simulink model "AERO2_LQR_OBSERVADOR"  (R2025b)
settings: Solver=ode1  StartTime=0.0  StopTime=inf  FixedStep=0.002  RelTol=1e-3  EnableMultiTasking=on
values from neighbouring files (symbols this model uses):
  A_modelo = [0 0 1 0 ... (first row only)    [AERO2_LQR_OBSERVADOR.m]
  B_modelo = [0 0 ... (first row only)    [AERO2_LQR_OBSERVADOR.m]
  beta = double(solucion.beta)    [AERO2_LQR_OBSERVADOR.m]
  C = [1 0 0 0 ... (first row only)    [AERO2_LQR_OBSERVADOR.m]
  D = [0 0 ... (first row only)    [AERO2_LQR_OBSERVADOR.m]
  K_lqr = lqr(A_modelo, B_modelo, Q, R)    [AERO2_LQR_OBSERVADOR.m]
  l = double(solucion.l)    [AERO2_LQR_OBSERVADOR.m]
  m = double(solucion.m)    [AERO2_LQR_OBSERVADOR.m]
undefined symbols (not defined in the file or in its folder): HIL, qc_get_step_size
libraries: quarc_library x7
settings Model: ExtModeTrigDuration=10000  Creator=CPB0  LastModifiedBy=CPB0
settings SolverCC: AlgebraicLoopSolver=TrustRegion  PositivePriorityOrder=on
settings DataIOCC: ReturnWorkspaceOutputs=off
settings DebuggingCC: UnconnectedInputMsg=warning  UnconnectedOutputMsg=warning  UnconnectedLineMsg=warning  ArithmeticOperatorsInVariantConditions=warning
settings ModelReferenceCC: EnableRefExpFcnMdlSchedulingChecks=on
settings SFSimCC: SimUseLocalCustomCode=off  CustomCodeUndefinedFunction=UseInterfaceOnly
settings RTWCC: SystemTargetFile=quarc_win64.tlc  TemplateMakefile=quarc_default_tmf  RTWUseLocalCustomCode=off  Toolchain=QUARC win64 | nmake (64-bit Windows)  BuildConfiguration=Faster Runs  GPUComputeCapability=3.5  Description=QUARC Win64 Target Using Toolchain
settings CodeAppCC: StateflowObjectComments=on
settings STFCustomTargetCC: SystemTargetFile=quarc_win64.tlc  TargetLangStandard=C99 (ISO)  UseToolchainInfoCompliant=on
settings GRTTargetCC: ExtMode=on  ExtModeMexFile=quarc_comm  ParMdlRefBuildCompliant=off  CompOptLevelCompliant=off  CombineOutputUpdateFcns=off  MatFileLogging=off  CPPClassGenCompliant=off  GRTInterface=on
settings ConfigComp: CovMetricSettings=dswe

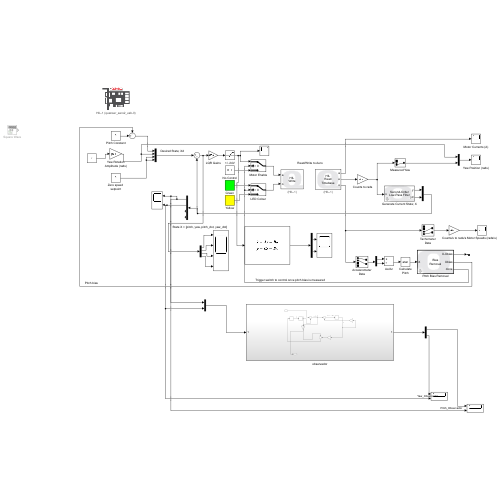
[thumbnail: Simulink's stored preview of the top-level diagram]
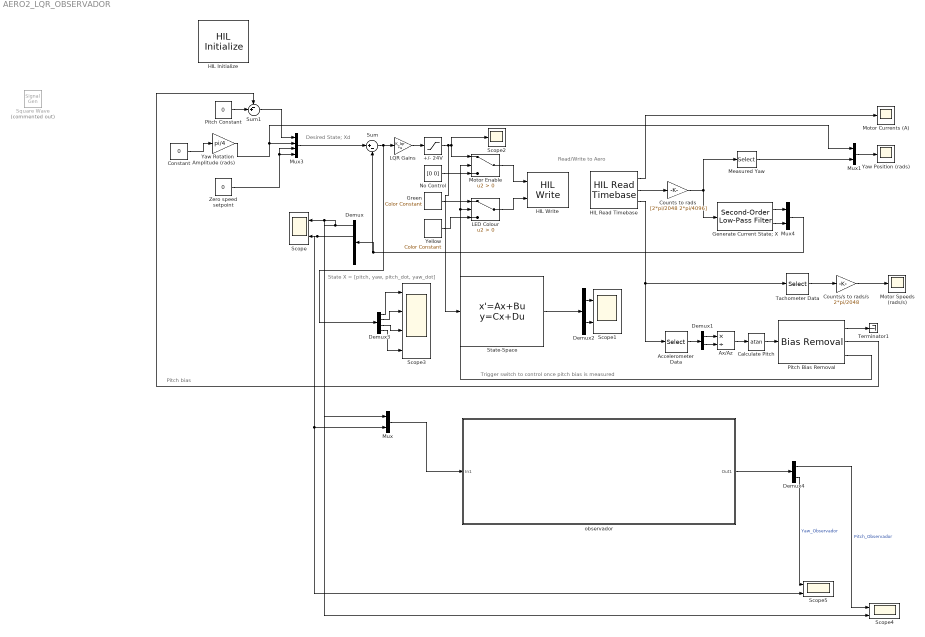
== system AERO2_LQR_OBSERVADOR ==
  note: Desired State; Xd
  note: Trigger switch to control once pitch bias is measured
  note: State X = [pitch, yaw, pitch_dot, yaw_dot]
  note: Pitch bias
  note: Read/Write to Aero
  +/- 24V : Saturate  UpperLimit=24  LowerLimit=-24
  Accelerometer Data : Selector  InputPortWidth=4  IndexOptions=Index vector (dialog)  Indices=[1 2]  OutputSizes=1
  Ax/Az : Product  Inputs=*/
  Calculate Pitch : Trigonometry  Operator=atan
  Constant : Constant  Value=0
  Counts to rads : Gain  Gain=[2*pi/2048 2*pi/4096]
  Counts/s to rads/s : Gain  Gain=2*pi/2048
  Demux : Demux
  Demux1 : Demux  Outputs=2
  Demux2 : Demux  Outputs=2
  Demux3 : Demux
  Demux4 : Demux  Outputs=2
  Generate Current State; X : quarc_library/Continuous/Second-Order Low-Pass Filter  params_source=Internal (dialog parameters)  input_width=50  input_zeta=0.8  input_init=0
  Green : quarc_library/Sources/Signals/Color Constant  color=[0 1 0]
      settings: SourceProductName=QUARC Targets
  HIL Initialize : quarc_library/Data Acquisition/Generic/Configuration/HIL Initialize  Priority=-99  object_name=HIL-1  board_type=quanser_aero2_usb  board_number=0  board_options=""  exclusive=off  active=off  hardware_clocks=[0]  clock_modes=[]  initial_clock_frequencies=[]  set_clock_params_at_start=off  set_clock_params_at_switch_in=off  set_clock_frequencies_at_start=off  set_clock_frequencies_at_switch_in=off  analog_input_channels=[0:1]  analog_input_configurations=[]  analog_input_maximums=3  analog_input_minimums=-3  set_analog_input_params_at_start=off  set_analog_input_params_at_switch_in=off  analog_output_channels=[0:1]  analog_output_maximums=24  analog_output_minimums=-24  initial_analog_outputs=[0]  final_analog_outputs=[0]  watchdog_analog_outputs=[0]  set_analog_output_params_at_start=off  set_analog_output_params_at_switch_in=off  set_analog_outputs_at_start=on  set_analog_outputs_at_switch_in=off  set_analog_outputs_at_terminate=on  set_analog_outputs_at_switch_out=off  set_analog_outputs_on_watchdog=on  digital_input_channels=[]  digital_output_channels=[0:1]  digital_output_configuration=[]  initial_digital_outputs=[1]  final_digital_outputs=[0]  watchdog_digital_outputs=[0]  set_digital_output_params_at_start=off  set_digital_output_params_at_switch_in=off  set_digital_outputs_at_start=on  set_digital_outputs_at_switch_in=off  set_digital_outputs_at_terminate=on  set_digital_outputs_at_switch_out=off  set_digital_outputs_on_watchdog=on  encoder_channels=[0:3]  quadrature=[4]  encoder_filter_frequency=[]  initial_encoder_counts=[0]  set_encoder_params_at_start=off  set_encoder_params_at_switch_in=off  set_encoder_counts_at_start=on  set_encoder_counts_at_switch_in=off  pwm_channels=[]  pwm_modes=[]  pwm_frequency=[]  pwm_configuration=[]  pwm_alignment=[]  pwm_polarity=[]  pwm_leading_deadband=[]  pwm_trailing_deadband=[]  initial_pwm_outputs=[]  final_pwm_outputs=[]  watchdog_pwm_outputs=[]  set_pwm_params_at_start=off  set_pwm_params_at_switch_in=off  set_pwm_outputs_at_start=off  set_pwm_outputs_at_switch_in=off  set_pwm_outputs_at_terminate=off  set_pwm_outputs_at_switch_out=off  set_pwm_outputs_on_watchdog=off  other_output_channels=[11000:11002]  initial_other_outputs=[0 1 0]  final_other_outputs=[1 0 0]  watchdog_other_outputs=[0 0 1]  set_other_outputs_at_start=on  set_other_outputs_at_switch_in=off  set_other_outputs_at_terminate=on  set_other_outputs_at_switch_out=off  set_other_outputs_on_watchdog=on
  HIL Read Timebase : quarc_library/Data Acquisition/Generic/Timebases/HIL Read Timebase  object_name=HIL-1  clock=0  analog_channels=[0:1]  encoder_channels=[2:3]  digital_channels=[]  other_channels=[4000 4002 14000 14001]  active=on  vector_output=on  data_type_mode=Inherit via back propagation  encoder_data_type=double  digital_data_type=boolean  overflow_mode=Error on overflow  samples_in_buffer=max(ceil(1/qc_get_step_size), 1)
  HIL Write : quarc_library/Data Acquisition/Generic/Immediate I//O/HIL Write  object_name=HIL-1  analog_channels=[0:1]  pwm_channels=[]  digital_channels=[]  other_channels=[11000:11002]  sample_time=-1  active=off  vector_input=on
  LED Colour : Switch  Criteria=u2 > Threshold  SaturateOnIntegerOverflow=off  InputSameDT=off
  LQR Gains : Gain  Gain=K_lqr  Multiplication=Matrix(K*u)
  Measured Yaw : Selector  InputPortWidth=2  IndexOptions=Index vector (dialog)  Indices=[2]  OutputSizes=1
  Motor Currents (A) : Scope
      settings: TimeSpan=20  ActiveDisplayYMinimum=-2.8562486027274758  ActiveDisplayYMaximum=2.8580371115582386  DataLoggingMaxPoints=10000  DataLoggingSaveFormat=Array
  Motor Enable : Switch  Criteria=u2 > Threshold  SaturateOnIntegerOverflow=off  InputSameDT=off
  Motor Speeds (rads/s) : Scope
      settings: TimeSpan=20  ActiveDisplayYMinimum=-539.65453579787618  ActiveDisplayYMaximum=527.86719058689664  DataLoggingMaxPoints=10000  DataLoggingSaveFormat=Array
  Mux : Mux  Inputs=2
  Mux1 : Mux  Inputs=2
  Mux3 : Mux
  Mux4 : Mux  Inputs=2
  No Control : Constant  Value=[0 0]
  Pitch Bias Removal : quarc_library/Discrete/Bias Removal  start_time=0  end_time=1  switch_id=0  sample_time=qc_get_step_size
      settings: SourceProductName=QUARC Targets
  Pitch Constant : Constant  Value=0
  Scope{,1,4..5} (4 alike) : Scope  NumInputPorts=2
      Scope settings: ActiveDisplayYMinimum=-0.063346011482274464  ActiveDisplayYMaximum=0.14008326949917518  DataLoggingVariableName=ScopeData2
      Scope1 settings: ActiveDisplayYMinimum=-186.67676145219883  ActiveDisplayYMaximum=36.029144431117452  DataLoggingVariableName=ScopeData3
      Scope4 settings: ActiveDisplayYMinimum=-1.6666209202121671  ActiveDisplayYMaximum=1.6178296829970562  DataLoggingVariableName=ScopeData7
      Scope5 settings: ActiveDisplayYMinimum=-0.81276536096715257  ActiveDisplayYMaximum=0.61965182279527964  DataLoggingVariableName=ScopeData8
  Scope2 : Scope
      settings: ActiveDisplayYMinimum=-42.75286877362997  ActiveDisplayYMaximum=41.423539651349842  DataLoggingVariableName=ScopeData5
  Scope3 : Scope  NumInputPorts=4
      settings: ActiveDisplayYMinimum=-1.5037000319110887  ActiveDisplayYMaximum=1.8470170140061124  DataLoggingVariableName=ScopeData6
  "Square Wave " : SignalGenerator  Commented=on  WaveForm=square  Frequency=0.1
  State-Space : StateSpace  A=A_modelo  B=B_modelo  C=C  D=D  InitialCondition=0
  Sum : Sum  Inputs=|+-
  Sum1 : Sum  Inputs=-+|
  Tachometer Data : Selector  InputPortWidth=4  IndexOptions=Index vector (dialog)  Indices=[3 4]  OutputSizes=1
  Terminator1 : Terminator
  Yaw Position (rads) : Scope
      settings: TimeSpan=20  ActiveDisplayYMinimum=-0.0042184471666855119  ActiveDisplayYMaximum=0.037966024500169615  DataLoggingMaxPoints=10000  DataLoggingVariableName=ScopeData4  DataLoggingSaveFormat=Array
  Yaw Rotation Amplitude (rads) : Gain  Gain=pi/4
  Yellow : quarc_library/Sources/Signals/Color Constant  color=[1 1 0]
      settings: SourceProductName=QUARC Targets
  Zero speed setpoint : Constant  Value=0
  observador : Subsystem
  wires:
  +/- 24V/1 -> State-Space/1, Scope2/1, Motor Enable/1
  Demux3/2 -> Scope3/2
  Green/1 -> LED Colour/1
  Pitch Constant/1 -> Sum1/2
  Tachometer Data/1 -> Counts/s to rads/s/1
  Demux1/1 -> Ax/Az/1
  Demux1/2 -> Ax/Az/2
  Pitch Bias Removal/2 -> Sum1/1
  Mux/1 -> observador/1(In1)
  Sum1/1 -> Mux3/1
  Mux4/1 -> Demux/1, Sum/2
  Constant/1 -> Yaw Rotation Amplitude (rads)/1
  Counts to rads/1 -> Measured Yaw/1, Generate Current State; X/1
  Calculate Pitch/1 -> Pitch Bias Removal/1
  Pitch Bias Removal/1 -> Terminator1/1
  Motor Enable/1 -> HIL Write/1
  Demux2/1 -> Scope1/1
  Sum/1 -> Demux3/1, LQR Gains/1
  Yellow/1 -> LED Colour/3
  No Control/1 -> Motor Enable/3
  HIL Read Timebase/1 -> Motor Currents (A)/1
  Demux/1 -> Scope4/2, Scope/1, Mux/1
  Pitch Bias Removal/3 -> Motor Enable/2, LED Colour/2
  Zero speed setpoint/1 -> Mux3/3, Mux3/4
  LQR Gains/1 -> +/- 24V/1
  Ax/Az/1 -> Calculate Pitch/1
  Generate Current State; X/1 -> Mux4/1
  Counts/s to rads/s/1 -> Motor Speeds (rads/s)/1
  Demux3/1 -> Scope3/1
  Mux1/1 -> Yaw Position (rads)/1
  LED Colour/1 -> HIL Write/2
  Generate Current State; X/2 -> Mux4/2
  Accelerometer Data/1 -> Demux1/1
  State-Space/1 -> Demux2/1
  Demux4/1 -> Scope4/1  "Pitch_Observador"
  Demux2/2 -> Scope1/2
  HIL Read Timebase/2 -> Counts to rads/1
  Measured Yaw/1 -> Mux1/2
  Yaw Rotation Amplitude (rads)/1 -> Mux3/2, Mux1/1
  Demux4/2 -> Scope5/1  "Yaw_Observador"
  Demux3/4 -> Scope3/4
  observador/1(Out1) -> Demux4/1
  HIL Read Timebase/3 -> Accelerometer Data/1, Tachometer Data/1
  Mux3/1 -> Sum/1
  Demux3/3 -> Scope3/3
  Demux/2 -> Scope5/2, Mux/2, Scope/2

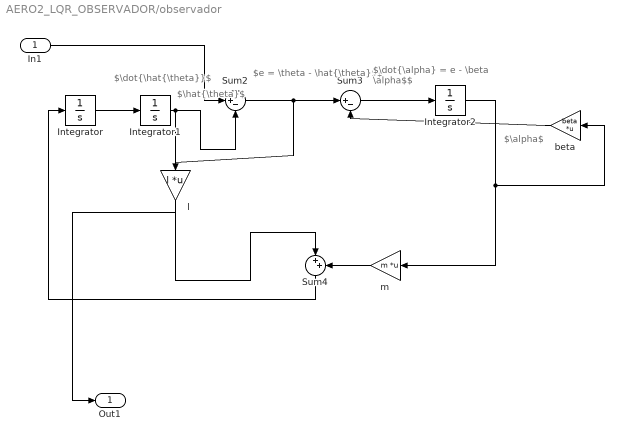
== system AERO2_LQR_OBSERVADOR/observador ==
  note: $\hat{\theta}$
  note: $\dot{\hat{\theta}}$
  note: $\alpha$
  note: $e = \theta - \hat{\theta}$$
  note: $\dot{\alpha} = e - \beta \alpha$$
  In1 : Inport
  Integrator : Integrator
  Integrator1 : Integrator
  Integrator2 : Integrator
  Sum2 : Sum  Inputs=|+-
  Sum3 : Sum  Inputs=|+-
  Sum4 : Sum  Inputs=|++
  beta : Gain  Gain=beta  Multiplication=Matrix(K*u)
  l : Gain  Gain=l  Multiplication=Matrix(K*u)
  m : Gain  Gain=m  Multiplication=Matrix(K*u)
  Out1 : Outport
  wires:
  beta/1 -> Sum3/2
  l/1 -> Sum4/1
  Integrator2/1 -> beta/1, m/1
  Sum4/1 -> Integrator/1
  Sum2/1 -> Sum3/1, l/1
  Integrator/1 -> Integrator1/1
  m/1 -> Sum4/2
  Integrator1/1 -> Out1/1, Sum2/2
  Sum3/1 -> Integrator2/1
  In1/1 -> Sum2/1
